simulink model "adqui"  (R2014b)
settings: Solver=ode45  StartTime=0.0  StopTime=300  RelTol=1e-3
libraries: opclib x4
settings Model: Creator=user  LastModifiedBy=user

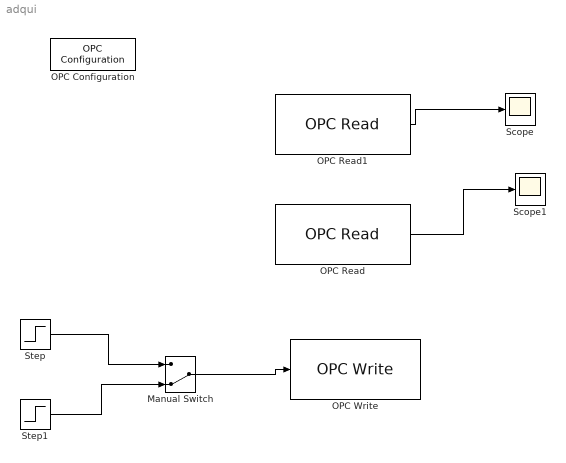
== system adqui ==
  Manual Switch : ManualSwitch  CurrentSetting=0
  OPC Configuration : opclib/OPC Configuration  opcServers=localhost/Kepware.KEPServerEX.V5/10  errMissingItems=Error  errReadWrite=Warn  errShutdown=Error  errRTViolation=Warn  rtEnable=on  speedup=1  showLatency=off  beingUsed=on
  OPC Read : opclib/OPC Read  serverHost=localhost  serverID=Kepware.KEPServerEX.V5  itemIDs=Channel1.Device1.Flujo  readMode=Synchronous (cache)  dataType=single  updateRate=0.5  showQual=off  showTS=off  tsMode=Seconds since start
  OPC Read1 : opclib/OPC Read  serverHost=localhost  serverID=Kepware.KEPServerEX.V5  itemIDs=Channel1.Device1.Presion  readMode=Synchronous (cache)  dataType=single  updateRate=0.5  showQual=off  showTS=off  tsMode=Seconds since start
  OPC Write : opclib/OPC Write  serverHost=localhost  serverID=Kepware.KEPServerEX.V5  itemIDs=Channel1.Device1.bomba  writeMode=Synchronous  updateRate=0
  Scope : Scope
      settings: YMin=-2  YMax=10
  Scope1 : Scope
      settings: YMin=-50  YMax=450  SaveName=flujo
  Step : Step  SampleTime=0
  Step1 : Step  After=0  SampleTime=0
  wires:
  OPC Read1/1 -> Scope/1
  OPC Read/1 -> Scope1/1
  Manual Switch/1 -> OPC Write/1
  Step/1 -> Manual Switch/1
  Step1/1 -> Manual Switch/2
